simulink model "exercise3_simulink"  (R2023b)
settings: Solver=FixedStepAuto  StartTime=0.0  StopTime=20  FixedStep=0.005  RelTol=1e-3
values from neighbouring files (symbols this model uses):
  F = flow    [call_RTO3.m]    (also in minCostFunction.m = x(1); nonlinearcon.m = x(1))
  kla = par(4)    [minCostFunction.m]    (also in nonlinearcon.m)
  sf = 10    [call_RTO3.m]    (also in minCostFunction.m = par(5); nonlinearcon.m = par(5))
  T = Temp    [call_RTO3.m]    (also in minCostFunction.m = x(2); nonlinearcon.m = x(2))
settings Model: Creator=s223446  LastModifiedBy=s223593
settings OptimizationCC: ReuseModelBlockBuffer=off
settings ModelReferenceCC: EnableRefExpFcnMdlSchedulingChecks=on

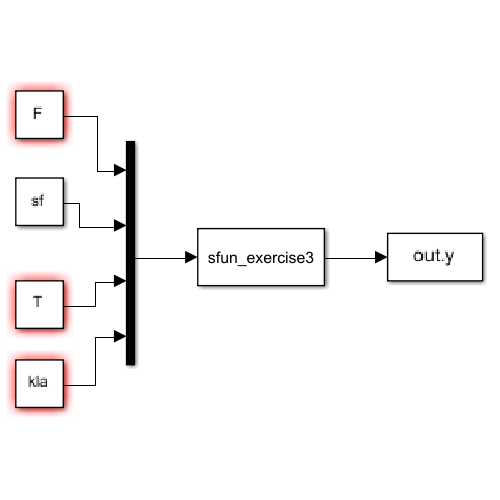
[thumbnail: Simulink's stored preview of the top-level diagram]
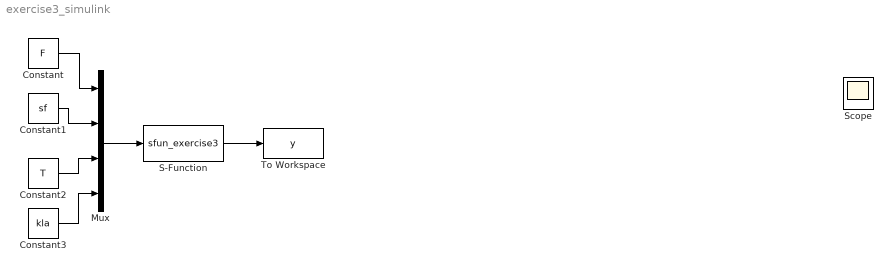
== system exercise3_simulink ==
  Constant : Constant  Value=F
  Constant1 : Constant  Value=sf
  Constant2 : Constant  Value=T
  Constant3 : Constant  Value=kla
  Mux : Mux
  S-Function : S-Function  FunctionName=sfun_exercise3  Parameters=xinit, par  SFunctionDeploymentMode=off  EnableBusSupport=off
  To Workspace : ToWorkspace  VariableName=y  SampleTime=-1
  Scope : Scope
  wires:
  Constant2/1 -> Mux/3
  Constant1/1 -> Mux/2
  Constant/1 -> Mux/1
  Mux/1 -> S-Function/1
  S-Function/1 -> To Workspace/1
  Constant3/1 -> Mux/4
